simulink model "chap1_7"  (R2022b)
settings: Solver=ode4  StartTime=0.0  StopTime=1  RelTol=1e-3  EnableMultiTasking=on
undefined symbols (not defined in the file or in its folder): chap1_7ctrl, chap1_7ctrl_Copy
settings Model: Creator=Train  LastModifiedBy=Train
settings SolverCC: AlgebraicLoopSolver=TrustRegion
settings DataIOCC: Decimation=100  SaveFormat=Array  SignalLoggingSaveFormat=ModelDataLogs  SaveOutput=off  SaveTime=off  ReturnWorkspaceOutputs=off
settings OptimizationCC: BlockReduction=off  BooleanDataType=off  InitFltsAndDblsToZero=on  LifeSpan=inf
settings DebuggingCC: SaveWithParameterizedLinksMsg=none  UnderspecifiedInitializationDetection=Classic  MergeDetectMultiDrivingBlocksExec=none  SignalResolutionControl=TryResolveAllWithWarning  MultiTaskDSMMsg=warning  MultiTaskCondExecSysMsg=none  FcnCallInpInsideContextMsg=warning  UnconnectedInputMsg=warning  UnconnectedOutputMsg=warning  UnconnectedLineMsg=warning  SFUnexpectedBacktrackingDiag=warning  SFNoUnconditionalDefaultTransitionDiag=warning  SFExecutionAtInitializationDiag=none  SFMachineParentedDataDiag=warning  ArithmeticOperatorsInVariantConditions=warning
settings HardwareCC: ProdBitPerPointer=32  ProdBitPerSizeT=32  ProdBitPerPtrDiffT=32  ProdLargestAtomicFloat=None  ProdIntDivRoundTo=Undefined  ProdEndianess=Unspecified  ProdWordSize=32  ProdHWDeviceType=32-bit Generic  TargetUnknown=on
settings ModelReferenceCC: PropagateSignalLabelsOutOfModel=off
settings CodeAppCC: StateflowObjectComments=on
settings GRTTargetCC: TargetFcnLib=ansi_tfl_tmw.mat  TargetLangStandard=C89/C90 (ANSI)  CombineOutputUpdateFcns=off  GRTInterface=on
settings ConfigComp: CovMetricSettings=dw  CovSaveCumulativeToWorkspaceVar=on  CovSaveSingleToWorkspaceVar=on

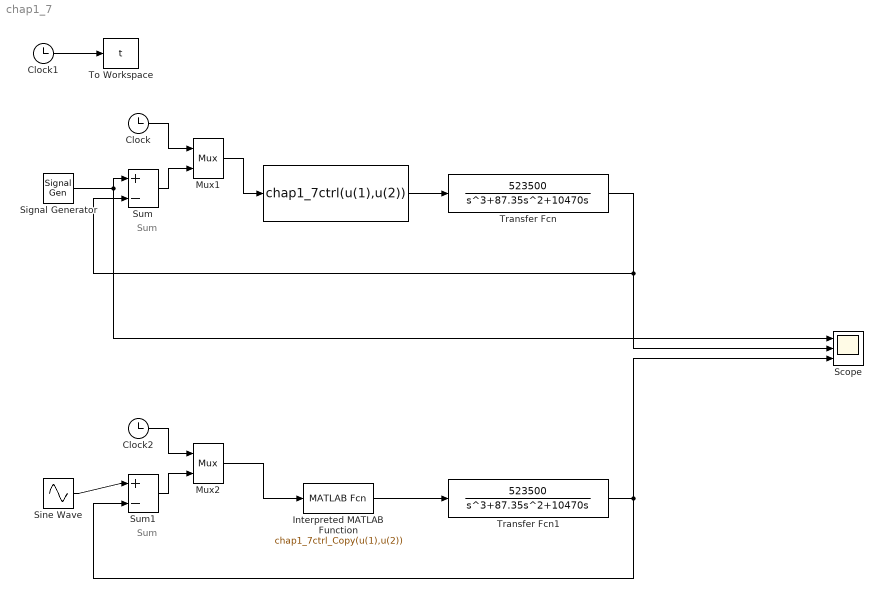
== system chap1_7 ==
  note: Sum
  note: Sum
  " " : MATLABFcn  MATLABFcn=chap1_7ctrl(u(1),u(2))
  Clock : Clock
  Clock1 : Clock
  Clock2 : Clock
  Interpreted MATLAB Function : MATLABFcn  MATLABFcn=chap1_7ctrl_Copy(u(1),u(2))
  Mux1 : Mux  Inputs=2
  Mux2 : Mux  Inputs=2
  Scope : Scope  NumInputPorts=3
  Signal Generator : SignalGenerator  Amplitude=0.05
  Sine Wave : Sin  Frequency=1*2*pi
  Sum : Sum  Inputs=|+-  InputSameDT=on  SaturateOnIntegerOverflow=on  OutDataTypeStr=Inherit: Same as first input
  Sum1 : Sum  Inputs=|+-  InputSameDT=on  SaturateOnIntegerOverflow=on  OutDataTypeStr=Inherit: Same as first input
  To Workspace : ToWorkspace  VariableName=t  SampleTime=-1
  Transfer Fcn : TransferFcn  Numerator=[523500]  Denominator=[1 87.35 10470 0]
  Transfer Fcn1 : TransferFcn  Numerator=[523500]  Denominator=[1 87.35 10470 0]
  wires:
  Transfer Fcn/1 -> Scope/2, Sum/2
  Signal Generator/1 -> Scope/1, Sum/1
  Clock/1 -> Mux1/1
  Sum/1 -> Mux1/2
  Mux1/1 -> " "/1
  " "/1 -> Transfer Fcn/1
  Clock1/1 -> To Workspace/1
  Sine Wave/1 -> Sum1/1
  Clock2/1 -> Mux2/1
  Mux2/1 -> Interpreted MATLAB Function/1
  Sum1/1 -> Mux2/2
  Transfer Fcn1/1 -> Sum1/2, Scope/3
  Interpreted MATLAB Function/1 -> Transfer Fcn1/1
